simulink model "Problem1_Malata"  (R2023b)
settings: Solver=VariableStepAuto  StartTime=0.0  StopTime=20  RelTol=1e-3
values from neighbouring files (symbols this model uses):
  G1_den = [1 0 0]    [Finals_Problem1_Malata.m]    (also in Problem2_Caldo_Comia_Malabanan.m)
  G1_num = [1]    [Finals_Problem1_Malata.m]    (also in Problem2_Caldo_Comia_Malabanan.m)
  G2_den = [1 1]    [Finals_Problem1_Malata.m]    (also in Problem2_Caldo_Comia_Malabanan.m)
  G2_num = [1]    [Finals_Problem1_Malata.m]    (also in Problem2_Caldo_Comia_Malabanan.m)
  G3_den = [1 0]    [Finals_Problem1_Malata.m]    (also in Problem2_Caldo_Comia_Malabanan.m)
  G3_num = [1]    [Finals_Problem1_Malata.m]    (also in Problem2_Caldo_Comia_Malabanan.m)
  H1_den = [1 0]    [Finals_Problem1_Malata.m]    (also in Problem2_Caldo_Comia_Malabanan.m)
  H1_num = [1]    [Finals_Problem1_Malata.m]    (also in Problem2_Caldo_Comia_Malabanan.m)
  H2_den = [1 -1]    [Finals_Problem1_Malata.m]    (also in Problem2_Caldo_Comia_Malabanan.m)
  H2_num = [1]    [Finals_Problem1_Malata.m]    (also in Problem2_Caldo_Comia_Malabanan.m)
  H3_den = [1 -2]    [Finals_Problem1_Malata.m]    (also in Problem2_Caldo_Comia_Malabanan.m)
  H3_num = [1]    [Finals_Problem1_Malata.m]    (also in Problem2_Caldo_Comia_Malabanan.m)
  TF_den = conv(TFG2G3H3_den,TFG1G2H1H2_den)    [Finals_Problem1_Malata.m]
  TF_num = conv(TFG2G3H3_num,TFG1G2H1H2_num)    [Finals_Problem1_Malata.m]
settings Model: Creator=Glenn  LastModifiedBy=Glenn

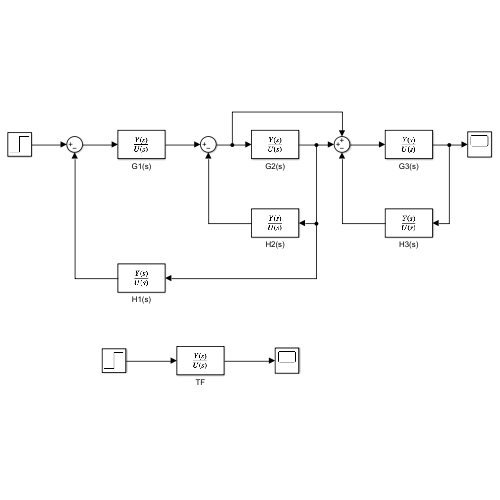
[thumbnail: Simulink's stored preview of the top-level diagram]
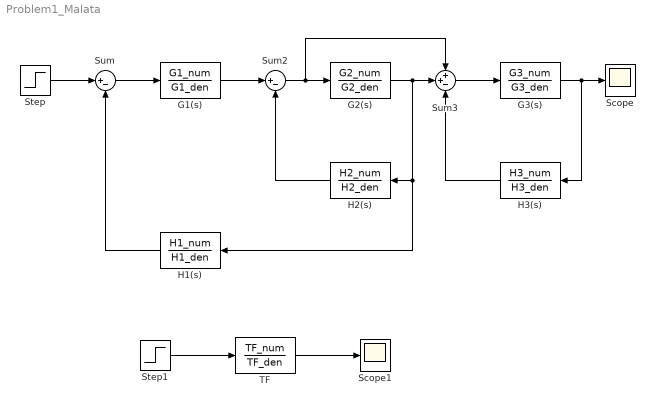
== system Problem1_Malata ==
  G1(s) : TransferFcn  Numerator=G1_num  Denominator=G1_den
  G2(s) : TransferFcn  Numerator=G2_num  Denominator=G2_den
  G3(s) : TransferFcn  Numerator=G3_num  Denominator=G3_den
  H1(s) : TransferFcn  Numerator=H1_num  Denominator=H1_den
  H2(s) : TransferFcn  Numerator=H2_num  Denominator=H2_den
  H3(s) : TransferFcn  Numerator=H3_num  Denominator=H3_den
  Scope : Scope
  Scope1 : Scope
  Step : Step  Time=0  SampleTime=0
  Step1 : Step  Time=0  SampleTime=0
  Sum : Sum  Inputs=|+-
  Sum2 : Sum  Inputs=|+-
  Sum3 : Sum  Inputs=++-
  TF : TransferFcn  Numerator=TF_num  Denominator=TF_den
  wires:
  Step/1 -> Sum/1
  Sum/1 -> G1(s)/1
  H1(s)/1 -> Sum/2
  G1(s)/1 -> Sum2/1
  Sum2/1 -> Sum3/1, G2(s)/1
  H2(s)/1 -> Sum2/2
  G2(s)/1 -> H1(s)/1, H2(s)/1, Sum3/2
  Sum3/1 -> G3(s)/1
  H3(s)/1 -> Sum3/3
  G3(s)/1 -> H3(s)/1, Scope/1
  Step1/1 -> TF/1
  TF/1 -> Scope1/1
